simulink model "Mondmission"  (R2015a)
settings: Solver=ode45  SolverMode=SingleTasking  StartTime=0.0  StopTime=5900  MaxStep=100  RelTol=1e-3
undefined symbols (not defined in the file): x0
settings Model: Creator=Ilja  LastModifiedBy=Daniel
settings OptimizationCC: BlockReduction=off  BooleanDataType=off
settings DebuggingCC: SaveWithParameterizedLinksMsg=none  UnderspecifiedInitializationDetection=Classic  MergeDetectMultiDrivingBlocksExec=none  SignalResolutionControl=TryResolveAllWithWarning
settings HardwareCC: TargetUnknown=on

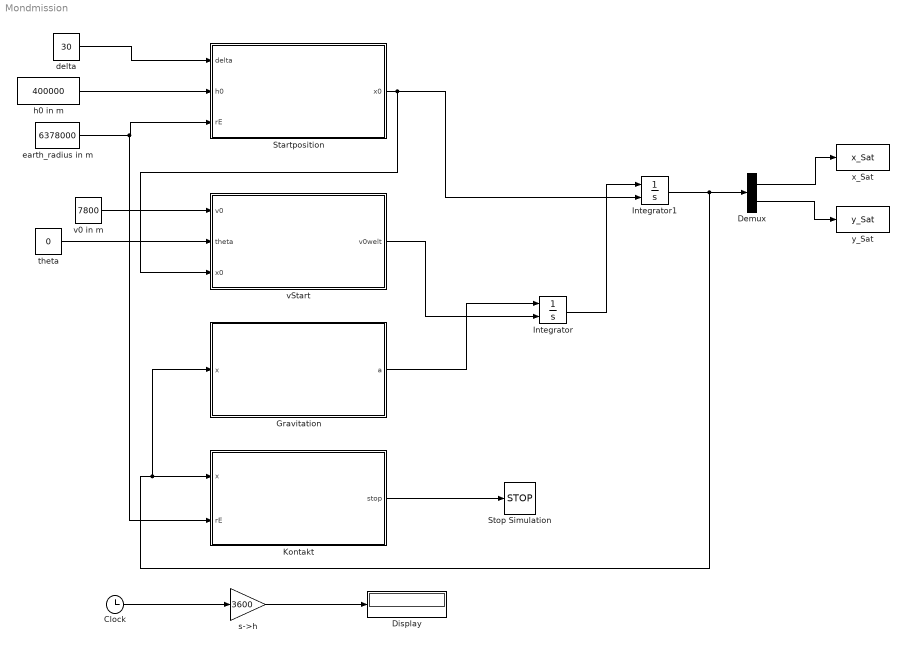
== system Mondmission ==
  Clock : Clock
  Demux : Demux  Outputs=2
  Display : Display
  Gravitation : MATLAB Function  TreatAsAtomicUnit=on
  Integrator : Integrator  InitialConditionSource=external  InitialCondition=x0
  Integrator1 : Integrator  InitialConditionSource=external
  Kontakt : MATLAB Function  TreatAsAtomicUnit=on
  Startposition : MATLAB Function  TreatAsAtomicUnit=on
  Stop Simulation : Stop
  delta : Constant  Value=30
  earth_radius in m : Constant  Value=6378000
  h0 in m : Constant  Value=400000
  s->h : Gain  Gain=3600
  theta : Constant  Value=0
  v0 in m : Constant  Value=7800
  vStart : MATLAB Function  TreatAsAtomicUnit=on
  x_Sat : ToWorkspace  VariableName=x_Sat  SampleTime=-1
  y_Sat : ToWorkspace  VariableName=y_Sat  SampleTime=-1
  wires:
  earth_radius in m/1 -> Kontakt/2(rE), Startposition/3(rE)
  delta/1 -> Startposition/1(delta)
  h0 in m/1 -> Startposition/2(h0)
  Startposition/1(x0) -> Integrator1/2, vStart/3(x0)
  theta/1 -> vStart/2(theta)
  v0 in m/1 -> vStart/1(v0)
  Kontakt/1(stop) -> Stop Simulation/1
  Clock/1 -> s->h/1
  s->h/1 -> Display/1
  Gravitation/1(a) -> Integrator/1
  Integrator/1 -> Integrator1/1
  vStart/1(v0welt) -> Integrator/2
  Integrator1/1 -> Gravitation/1(x), Kontakt/1(x), Demux/1
  Demux/1 -> x_Sat/1
  Demux/2 -> y_Sat/1

== matlab function Mondmission/vStart ==
  data: v0 input; theta input; x0 input; v0welt output
function v0welt = vStart(v0, theta, x0)
    thetaBog = theta * pi/180; %Umrechnung Bogenmaß
    n = x0/norm(x0);
    t = [n(2);-n(1)];  
    vn = sin(thetaBog) * v0;
    vt = cos(thetaBog) * v0;
    v0welt = vn * n + vt * t;

== matlab function Mondmission/Startposition ==
  data: delta input; x0 output; h0 input; rE input
function x0 = Startposition(delta, h0, rE)
    deltaBog = delta * pi/180; %Umrechnung Bogenmaß
    x0 = [cos(deltaBog)*(h0+rE);sin(deltaBog)*(h0+rE)];

== matlab function Mondmission/Gravitation ==
  data: x input; a output
function a = Gravitaion(x)
    G = 66.743*10^-12;
    mE = 5.9736*10^24;
    mM = 7.3480*10^22;
    xM = [0; -380000000];
    m = xM - x % Mondkomponente
    
    aE = G * mE * (-x/norm(x)) / (norm(x)^2); % Newtonsches Gravitaionsgesetz
    aG = G * mM * (-m/norm(m)) / (norm(m)^2);
    
    a = aE + aM;

== matlab function Mondmission/Kontakt ==
  data: x input; stop output; rE input
function stop = Kontakt(x, rE)
    stop = 0;
    if norm(x) <= rE
        stop = 1;
    end
